simulink model "modelo13_8"  (R2020a)
settings: Solver=ode45  StartTime=0.0  StopTime=0.08  RelTol=1e-3  EnableMultiTasking=on
values from neighbouring files (symbols this model uses):
  cequa = 0    [RotinaCurtoCircuito.m]    (also in RotinaCurtoCircuitoCompacto.m; RotinaCurtoCircuitoCompleta.m; RotinaCurtoCircuitoT2F_Trifasico.m; TesteArtigo1.m)
  le = 1e-10    [RotinaCurtoCircuito.m]    (also in RotinaCurtoCircuitoCompacto.m; RotinaCurtoCircuitoCompleta.m; RotinaCurtoCircuitoT2F_Trifasico.m; TesteArtigo1.m)
  NRE = 1e-12    [RotinaCurtoCircuito.m]    (also in RotinaCurtoCircuitoCompacto.m; RotinaCurtoCircuitoCompleta.m; RotinaCurtoCircuitoT2F_Trifasico.m; TesteArtigo1.m)
  rtc = Resistencias    (= 10)    [CalculoCircuitoTreinamento.m]    (also in RotinaCurtoCircuito.m; RotinaCurtoCircuitoCompacto.m; RotinaCurtoCircuitoCompleta.m; RotinaCurtoCircuitoT2F_Trifasico.m)
  rti = Resistencias    (= 10)    [CalculoCircuitoTreinamento.m]    (also in RotinaCurtoCircuito.m; RotinaCurtoCircuitoCompacto.m; RotinaCurtoCircuitoCompleta.m; RotinaCurtoCircuitoT2F_Trifasico.m)
undefined symbols (not defined in the file or in its folder): C_matrix, D11, Delta, L_matrix, R_matrix
libraries: powerlib x19
settings Model: Creator=laris  LastModifiedBy=Usuario
settings DataIOCC: LimitDataPoints=on  SaveFormat=Array  ReturnWorkspaceOutputs=off
settings OptimizationCC: LifeSpan=inf
settings DebuggingCC: SFUnexpectedBacktrackingDiag=warning  SFNoUnconditionalDefaultTransitionDiag=warning  SFExecutionAtInitializationDiag=none  ArithmeticOperatorsInVariantConditions=warning
settings HardwareCC: ProdBitPerPointer=32  ProdBitPerSizeT=32  ProdBitPerPtrDiffT=32  ProdLargestAtomicFloat=None  ProdIntDivRoundTo=Undefined  ProdEndianess=Unspecified  ProdWordSize=32  ProdHWDeviceType=32-bit Generic
settings ModelReferenceCC: PropagateSignalLabelsOutOfModel=off
settings SFSimCC: SimUseLocalCustomCode=off  CustomCodeUndefinedFunction=UseInterfaceOnly
settings RTWCC: RTWUseLocalCustomCode=off
settings CodeAppCC: StateflowObjectComments=on
settings GRTTargetCC: TargetLangStandard=C89/C90 (ANSI)
settings ConfigComp: CovMetricSettings=dw  CovHtmlReporting=on  CovSaveCumulativeToWorkspaceVar=on  CovSaveSingleToWorkspaceVar=on  CovExternalEMLEnable=off
settings SimscapeCC: SimscapeNormalizeSystem=off

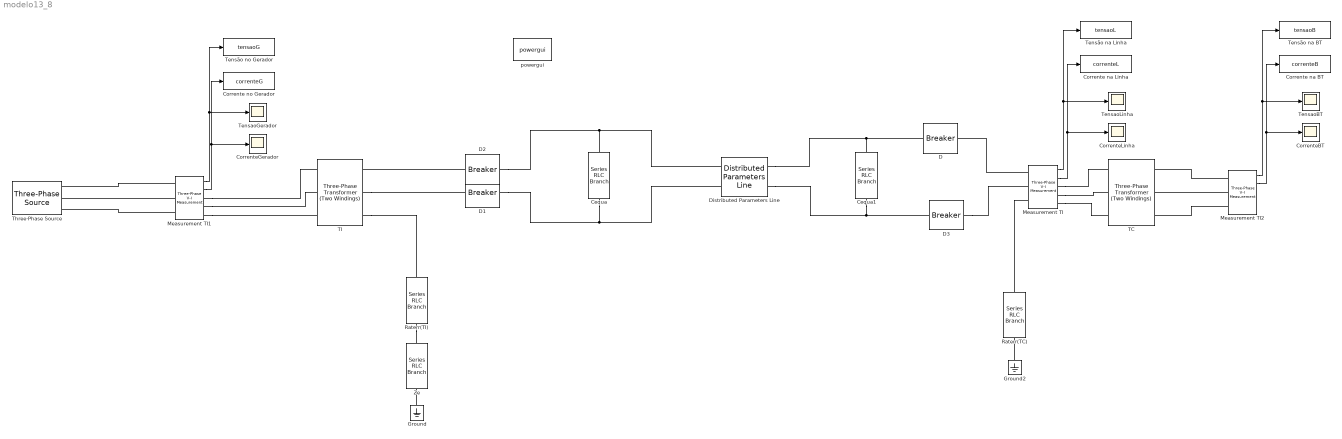
== system modelo13_8 ==
  Cequa : powerlib/Elements/Series RLC Branch  LConnTagsString=__new0  RConnTagsString=__new0  BranchType=C  Resistance=1  Inductance=1e-3  SetiL0=off  InitialCurrent=0  Capacitance=cequa/2  Setx0=off  InitialVoltage=0  Measurements=None
  Cequa1 : powerlib/Elements/Series RLC Branch  LConnTagsString=__new0  RConnTagsString=__new0  BranchType=C  Resistance=1  Inductance=1e-3  SetiL0=off  InitialCurrent=0  Capacitance=cequa/2  Setx0=off  InitialVoltage=0  Measurements=None
  Corrente na BT : ToWorkspace  VariableName=correnteB  SampleTime=-1
  Corrente na Linha : ToWorkspace  VariableName=correnteL  SampleTime=-1
  "Corrente no Gerador " : ToWorkspace  VariableName=correnteG  SampleTime=-1
  CorrenteBT : Scope
  CorrenteGerador : Scope
  CorrenteLinha : Scope
  D : powerlib/Elements/Breaker  InitialState=1  SwitchingTimes=[1 ]  External=off  BreakerResistance=0.01  SnubberResistance=1e6  SnubberCapacitance=inf  Measurements=None  MoreParameters=on  NoBreakLoop=off
  D1 : powerlib/Elements/Breaker  InitialState=1  SwitchingTimes=[1 ]  External=off  BreakerResistance=0.01  SnubberResistance=1e6  SnubberCapacitance=inf  Measurements=None  MoreParameters=on  NoBreakLoop=off
  D2 : powerlib/Elements/Breaker  InitialState=0  SwitchingTimes=[1 ]  External=off  BreakerResistance=0.01  SnubberResistance=1e6  SnubberCapacitance=inf  Measurements=None  MoreParameters=on  NoBreakLoop=off
  D3 : powerlib/Elements/Breaker  InitialState=0  SwitchingTimes=[1 ]  External=off  BreakerResistance=0.01  SnubberResistance=1e6  SnubberCapacitance=inf  Measurements=None  MoreParameters=on  NoBreakLoop=off
  Distributed Parameters Line : powerlib/Elements/Distributed Parameters Line  Phases=2  Frequency=60  Resistance=R_matrix  Inductance=L_matrix  Capacitance=C_matrix  Length=d  x1=[1842.29848951702 34234.0705333129;376.991118430775 376.991118430775;0.98605198067235 -2.10219907004305]  x2=[1842.80518551664 34235.6839412644;376.991118430775 376.991118430775;0.985411759712884 -2.10224172771747]  x3=[4.95847483803439 39.1920615884785;376.991118430775 376.991118430775;0.946493944067575 -2.11204491628235]  x4=[4.9579539605154 39.2025372728194;376.991118430775 376.991118430775;1.01722811542495 -2.10224165111392]  x5=2.60584073245773e-05  V1=[1842 3.423e+04;377 377;0.9861 -2.102]  V2=[1843 3.424e+04;377 377;0.9854 -2.102]  I1=[4.958 39.19;377 377;0.9465 -2.112]  I2=[4.958 39.2;377 377;1.017 -2.102]  nHarmo=1  Measurements=None
  Ground : powerlib/Elements/Ground  LConnTagsString=a
  Ground2 : powerlib/Elements/Ground  LConnTagsString=a
  Measurement TI : powerlib/Measurements/Three-Phase V-I Measurement  VoltageMeasurement=phase-to-phase  SetLabelV=off  LabelV=Vabc  Vpu=off  VpuLL=off  CurrentMeasurement=yes  SetLabelI=off  LabelI=Iabc  Ipu=off  Pbase=100e6  Vbase=500e3  OutputType=Magnitude  PhasorSimulation=off  PSBequivalent=0
  Measurement TI1 : powerlib/Measurements/Three-Phase V-I Measurement  VoltageMeasurement=phase-to-phase  SetLabelV=off  LabelV=Vabc  Vpu=off  VpuLL=off  CurrentMeasurement=yes  SetLabelI=off  LabelI=Iabc  Ipu=off  Pbase=100e6  Vbase=500e3  OutputType=Magnitude  PhasorSimulation=off  PSBequivalent=0
  Measurement TI2 : powerlib/Measurements/Three-Phase V-I Measurement  VoltageMeasurement=phase-to-phase  SetLabelV=off  LabelV=Vabc  Vpu=off  VpuLL=off  CurrentMeasurement=yes  SetLabelI=off  LabelI=Iabc  Ipu=off  Pbase=100e6  Vbase=500e3  OutputType=Magnitude  PhasorSimulation=off  PSBequivalent=0
  Raterr(TC) : powerlib/Elements/Series RLC Branch  LConnTagsString=__new0  RConnTagsString=__new0  BranchType=R  Resistance=rtc  Inductance=0  SetiL0=off  InitialCurrent=0  Capacitance=1e-6  Setx0=off  InitialVoltage=0  Measurements=None
  Raterr(TI) : powerlib/Elements/Series RLC Branch  LConnTagsString=__new0  RConnTagsString=__new0  BranchType=R  Resistance=rti  Inductance=0  SetiL0=off  InitialCurrent=0  Capacitance=1e-6  Setx0=off  InitialVoltage=0  Measurements=None
  TC : powerlib/Elements/Three-Phase Transformer (Two Windings)  Winding1Connection=Delta (D11)  Winding2Connection=Yg  CoreType=Three single-phase transformers  SetSaturation=on  Hysteresis=off  DataFile='hysteresis'  SetInitialFlux=off  Measurements=None  UNITS=pu  NominalPower=[75e3 , 60]  Winding1=[13800 0.0312 0.031331]  Winding2=[220 0.031199 0.031331]  Rm=789.473064  Lm=525.63  L0=0.50001  Saturation=[0,0 ; 0.00149, 0.701;0.00392, 0.810; 0.00793,0.907; 0.01539,1.00; 0.02935, 1.1; 0.06018, 1.209]  InitialFluxes=[0.581641452542793 -0.0178573892400959 -0.563784063302697]  BreakLoop=off  DiscreteSolver=Trapezoidal iterative  DataType=off  TransfoNumber=1
  TI : powerlib/Elements/Three-Phase Transformer (Two Windings)  Winding1Connection=Delta (D11)  Winding2Connection=Y  CoreType=Three single-phase transformers  SetSaturation=off  Hysteresis=off  DataFile='hysteresis'  SetInitialFlux=off  Measurements=None  UNITS=pu  NominalPower=[120e3 , 60 ]  Winding1=[13800 0.0048119 0.018511]  Winding2=[13800 0.0048119 0.018511]  Rm=1.730769230769231e+03  Lm=40.010686750359440  L0=0.5  Saturation=[0 0;0.0012545 0.01913;0.52272 0.024231]  InitialFluxes=[0.66023 -0.66023 0.5777]  BreakLoop=off  DiscreteSolver=Trapezoidal iterative  DataType=off  TransfoNumber=1
  TensaoBT : Scope
  TensaoGerador : Scope
  TensaoLinha : Scope
  Tensão na BT : ToWorkspace  VariableName=tensaoB  SampleTime=-1
  Tensão na Linha : ToWorkspace  VariableName=tensaoL  SampleTime=-1
  Tensão no Gerador : ToWorkspace  VariableName=tensaoG  SampleTime=-1
  Three-Phase Source : powerlib/Electrical Sources/Three-Phase Source  InternalConnection=Yg  VoltagePhases=off  Voltage=13.8e3  PhaseAngle=0  Voltage_phases=[25e3 25e3 25e3]/sqrt(3)  PhaseAngles_phases=[0 -120 +120]  Frequency=60  NonIdealSource=on  SpecifyImpedance=on  Resistance=0.8929  Inductance=16.58e-3  ShortCircuitLevel=120e6  BaseVoltage=15e3  XRratio=7  BusType=swing  Pref=10e3  Qref=0  Prefabc=[10e3, 10e3, 10e3]  Qrefabc=[0, 0, 0]  Qmin=-inf  Qmax=inf
  Ze : powerlib/Elements/Series RLC Branch  LConnTagsString=__new0  RConnTagsString=__new0  BranchType=RL  Resistance=NRE  Inductance=le  SetiL0=off  InitialCurrent=0  Capacitance=le  Setx0=off  InitialVoltage=0  Measurements=None
  powergui : powerlib/powergui  Priority=1  SimulationMode=Continuous  SampleTime=50e-6  frequency=60  Iterations=50  frequencyindice=60  Pbase=100e6  ErrMax=1e-4  UnitsV=kV  UnitsW=MW  buscounter=0  FunctionMessages=off  echomessages=off  EnableUseOfTLC=off  CurrentSourceSwitches=off  DisableSnubberDevices=off  DisableRonSwitches=off  DisableVfSwitches=off  DisplayEquations=off  AutomaticDiscreteSolvers=off  SolverType=Tustin/Backward Euler (TBE)  Interpol=off  ExternalGateDelay=off  methode=off  Ts=100  x0status=blocks  SPID=on  SwTol=0  HookPort=off  NonlinearTolerance=1e-4  nMaxIteration=100  ContinueOnMaxIteration=off  RestoreLinks=warning  ResistiveCurrentMeasurement=off  Frange=[0:2:500]  Ylog=off  Xlog=on  ShowGrid=off  save=off  variable=ZData  structure=0  ZoomFFT=off  StartTime=0.0  cycles=1  DisplayStyle=1  fundamental=60  FreqAxis=off  MaxFrequency=1000  frequencyindicesteady=1  RmsSteady=1  display=off
  wires:
  Measurement TI2/1 -> TensaoBT/1, Tensão na BT/1
  Measurement TI1/2 -> CorrenteGerador/1, "Corrente no Gerador "/1
  Measurement TI1/1 -> TensaoGerador/1, Tensão no Gerador/1
  Measurement TI/1 -> TensaoLinha/1, Tensão na Linha/1
  Measurement TI/2 -> CorrenteLinha/1, Corrente na Linha/1
  Measurement TI2/2 -> CorrenteBT/1, Corrente na BT/1
  connections:
  Distributed Parameters Line/RConn2 -- Cequa1/RConn1 -- D3/LConn1
  D/LConn1 -- Cequa1/LConn1 -- Distributed Parameters Line/RConn1
  Measurement TI/RConn1 -- TC/LConn1
  Measurement TI/RConn2 -- TC/LConn2
  Measurement TI/RConn3 -- TC/LConn3
  D2/LConn1 -- TI/RConn1
  Cequa/RConn1 -- D1/RConn1 -- Distributed Parameters Line/LConn2
  TI/RConn3 -- Raterr(TI)/LConn1
  Measurement TI/LConn3 -- Raterr(TC)/RConn1
  Raterr(TI)/RConn1 -- Ze/LConn1
  Ground/LConn1 -- Ze/RConn1
  Ground2/LConn1 -- Raterr(TC)/LConn1
  Measurement TI/LConn1 -- D/RConn1
  TI/RConn2 -- D1/LConn1
  D2/RConn1 -- Cequa/LConn1 -- Distributed Parameters Line/LConn1
  D3/RConn1 -- Measurement TI/LConn2
  Measurement TI1/LConn3 -- Three-Phase Source/RConn3
  Measurement TI1/LConn2 -- Three-Phase Source/RConn2
  Measurement TI1/LConn1 -- Three-Phase Source/RConn1
  Measurement TI1/RConn2 -- TI/LConn2
  Measurement TI1/RConn3 -- TI/LConn3
  Measurement TI1/RConn1 -- TI/LConn1
  Measurement TI2/LConn2 -- TC/RConn2
  Measurement TI2/LConn1 -- TC/RConn1
  Measurement TI2/LConn3 -- TC/RConn3
